simulink model "RI_RL_PI_ZPK"  (R2013b)
settings: Solver=ode45  StartTime=0.0  StopTime=25*L/R  MaxStep=tau/100  RelTol=1e-3
InitFcn:
  | % Modellparaméterek
  | R = 250e-3;
  | L = 10e-3;
  | Psi_0 = 0.5e-3;
  | 
  | i_0 = 0;
  | theta_0 = 0;
  | 
  | % Rendszerparaméterek
  | K = 1/R;
  | tau = L/R;
libraries: RI_MK x4, simulink x1
settings Model: Creator=Szalay  LastModifiedBy=Szalay

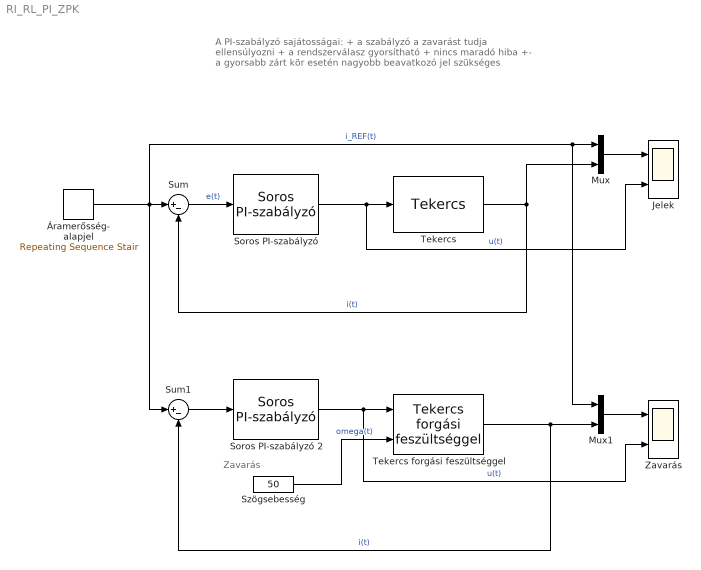
== system RI_RL_PI_ZPK ==
  note: A PI-szabályzó sajátosságai:
      | + a szabályzó a zavarást tudja ellensúlyozni
      | + a rendszerválasz gyorsítható
      | + nincs maradó hiba
      | +- a gyorsabb zárt kör esetén nagyobb beavatkozó jel szükséges
  note: Zavarás
  Jelek : Scope  NumInputPorts=2
      settings: ShowLegends=on  TimeRange=1  YMin=-0.4~-0.25  YMax=0.3~0.25
  Mux : Mux  Inputs=2
  Mux1 : Mux  Inputs=2
  Soros PI-szabályzó : RI_MK/Soros PI-szabályzó  K_PI=1/(1/R) * 25  T_I=L/R
  Soros PI-szabályzó 2 : RI_MK/Soros PI-szabályzó  K_PI=1/(1/R) * 10  T_I=L/R
  Sum : Sum  Inputs=|+-
  Sum1 : Sum  Inputs=|+-
  Szögsebesség : Constant  Value=50
  Tekercs : RI_MK/Tekercs  R=R  L=L  i_0=0
  Tekercs forgási feszültséggel : RI_MK/Tekercs forgási feszültséggel  R=R  L=L  Psi_0=Psi_0  i_0=i_0  theta_0=theta_0
  Zavarás : Scope  NumInputPorts=2
      settings: ShowLegends=on  YMin=-5~-5  YMax=5~5
  Áramerősség- alapjel : simulink/Sources/Repeating Sequence Stair  OutValues=[300, 100, -400, 200, -100]*1e-3  tsamp=L/R*5  OutMin=[]  OutMax=[]  OutDataTypeStr=double  OutputDataTypeScalingMode=double  OutDataType=fixdt(0,8)  ConRadixGroup=Best Precision: Vector-wise  OutScaling=2^-12
  wires:
  Mux/1 -> Jelek/1
  Tekercs/1 -> Sum/2, Mux/2  "i(t)"
  Mux1/1 -> Zavarás/1
  Szögsebesség/1 -> Tekercs forgási feszültséggel/2  "omega(t)"
  Soros PI-szabályzó 2/1 -> Zavarás/2, Tekercs forgási feszültséggel/1  "u(t)"
  Áramerősség- alapjel/1 -> Mux1/1, Mux/1, Sum/1, Sum1/1  "i_REF(t)"
  Tekercs forgási feszültséggel/1 -> Sum1/2, Mux1/2  "i(t)"
  Sum1/1 -> Soros PI-szabályzó 2/1
  Soros PI-szabályzó/1 -> Jelek/2, Tekercs/1  "u(t)"
  Sum/1 -> Soros PI-szabályzó/1  "e(t)"
